simulink model "PMSM_CCSMPC_ClosedLoop"  (R2025b)
settings: Solver=ode3  StartTime=0.0  StopTime=0.4  FixedStep=1e-6  RelTol=1e-3
PreLoadFcn:
  | run('params_pmsm_inverter')
undefined symbols (not defined in the file or in its folder): Iq_max, J, Ld_hat, Lq_hat, pp, PsiPM_hat, Rs_hat, Ts_ctrl, Ts_sim, Vdc
libraries: nesl_utility x13, fl_lib x8, ee_lib x8, simulink x1, slpidlib x1
(part 1 of 2)
settings Model: Creator=Harish  LastModifiedBy=Harish

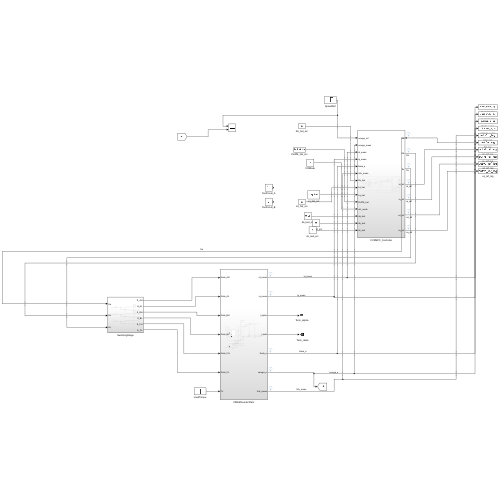
[thumbnail: Simulink's stored preview of the top-level diagram]
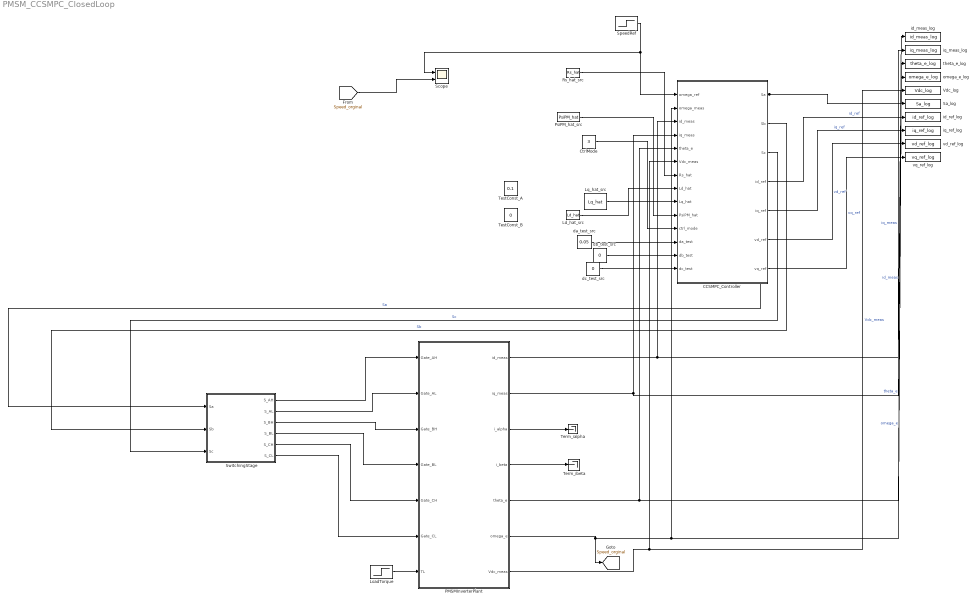
== system PMSM_CCSMPC_ClosedLoop ==
  CCSMPC_Controller : Subsystem
  CtrlMode : Constant  Value=3  OutDataTypeStr=uint8
  Ld_hat_src : Constant  Value=Ld_hat
  LoadTorque : Step  Time=0.25  After=0.05  SampleTime=0
  Lq_hat_src : Constant  Value=Lq_hat
  PMSMInverterPlant : Subsystem
  PsiPM_hat_src : Constant  Value=PsiPM_hat
  Rs_hat_src : Constant  Value=Rs_hat
  Sa_log : ToWorkspace  VariableName=Sa_log  SaveFormat=Timeseries  SampleTime=-1
  Scope : Scope  NumInputPorts=2
      settings: ActiveDisplayYMinimum=-24.999999999999993  ActiveDisplayYMaximum=225
  SpeedRef : Step  Time=0.05  After=200  SampleTime=0
  SwitchingStage : Subsystem
  Term_ialpha : Terminator
  Term_ibeta : Terminator
  TestConst_A : Constant  Value=0.1
  TestConst_B : Constant  Value=0
  Vdc_log : ToWorkspace  VariableName=Vdc_log  SaveFormat=Timeseries  SampleTime=-1
  da_test_src : Constant  Value=0.05
  db_test_src : Constant  Value=0
  dc_test_src : Constant  Value=0
  id_meas_log : ToWorkspace  VariableName=id_meas_log  SaveFormat=Timeseries  SampleTime=-1
  id_ref_log : ToWorkspace  VariableName=id_ref_log  SaveFormat=Timeseries  SampleTime=-1
  iq_meas_log : ToWorkspace  VariableName=iq_meas_log  SaveFormat=Timeseries  SampleTime=-1
  iq_ref_log : ToWorkspace  VariableName=iq_ref_log  SaveFormat=Timeseries  SampleTime=-1
  omega_e_log : ToWorkspace  VariableName=omega_e_log  SaveFormat=Timeseries  SampleTime=-1
  theta_e_log : ToWorkspace  VariableName=theta_e_log  SaveFormat=Timeseries  SampleTime=-1
  vd_ref_log : ToWorkspace  VariableName=vd_ref_log  SaveFormat=Timeseries  SampleTime=-1
  vq_ref_log : ToWorkspace  VariableName=vq_ref_log  SaveFormat=Timeseries  SampleTime=-1
  tag scope: Speed_orginal=global
  wires:
  SpeedRef/1 -> Scope/1, CCSMPC_Controller/1(omega_ref)
  Rs_hat_src/1 -> CCSMPC_Controller/7(Rs_hat)
  Ld_hat_src/1 -> CCSMPC_Controller/8(Ld_hat)
  Lq_hat_src/1 -> CCSMPC_Controller/9(Lq_hat)
  PsiPM_hat_src/1 -> CCSMPC_Controller/10(PsiPM_hat)
  CtrlMode/1 -> CCSMPC_Controller/11(ctrl_mode)
  PMSMInverterPlant/6(omega_e) -> [Speed_orginal], CCSMPC_Controller/2(omega_meas), omega_e_log/1  "omega_e"
  PMSMInverterPlant/1(id_meas) -> id_meas_log/1, CCSMPC_Controller/3(id_meas)  "id_meas"
  PMSMInverterPlant/2(iq_meas) -> iq_meas_log/1, CCSMPC_Controller/4(iq_meas)  "iq_meas"
  PMSMInverterPlant/5(theta_e) -> theta_e_log/1, CCSMPC_Controller/5(theta_e)  "theta_e"
  PMSMInverterPlant/7(Vdc_meas) -> CCSMPC_Controller/6(Vdc_meas), Vdc_log/1  "Vdc_meas"
  CCSMPC_Controller/1(Sa) -> SwitchingStage/1(Sa), Sa_log/1  "Sa"
  CCSMPC_Controller/2(Sb) -> SwitchingStage/2(Sb)  "Sb"
  CCSMPC_Controller/3(Sc) -> SwitchingStage/3(Sc)  "Sc"
  SwitchingStage/1(S_AH) -> PMSMInverterPlant/1(Gate_AH)
  SwitchingStage/2(S_AL) -> PMSMInverterPlant/2(Gate_AL)
  SwitchingStage/3(S_BH) -> PMSMInverterPlant/3(Gate_BH)
  SwitchingStage/4(S_BL) -> PMSMInverterPlant/4(Gate_BL)
  SwitchingStage/5(S_CH) -> PMSMInverterPlant/5(Gate_CH)
  SwitchingStage/6(S_CL) -> PMSMInverterPlant/6(Gate_CL)
  LoadTorque/1 -> PMSMInverterPlant/7(TL)
  CCSMPC_Controller/4(id_ref) -> id_ref_log/1  "id_ref"
  CCSMPC_Controller/5(iq_ref) -> iq_ref_log/1  "iq_ref"
  CCSMPC_Controller/6(vd_ref) -> vd_ref_log/1  "vd_ref"
  CCSMPC_Controller/7(vq_ref) -> vq_ref_log/1  "vq_ref"
  PMSMInverterPlant/3(i_alpha) -> Term_ialpha/1
  PMSMInverterPlant/4(i_beta) -> Term_ibeta/1
  db_test_src/1 -> CCSMPC_Controller/13(db_test)
  dc_test_src/1 -> CCSMPC_Controller/14(dc_test)
  da_test_src/1 -> CCSMPC_Controller/12(da_test)
  [Speed_orginal] -> Scope/2

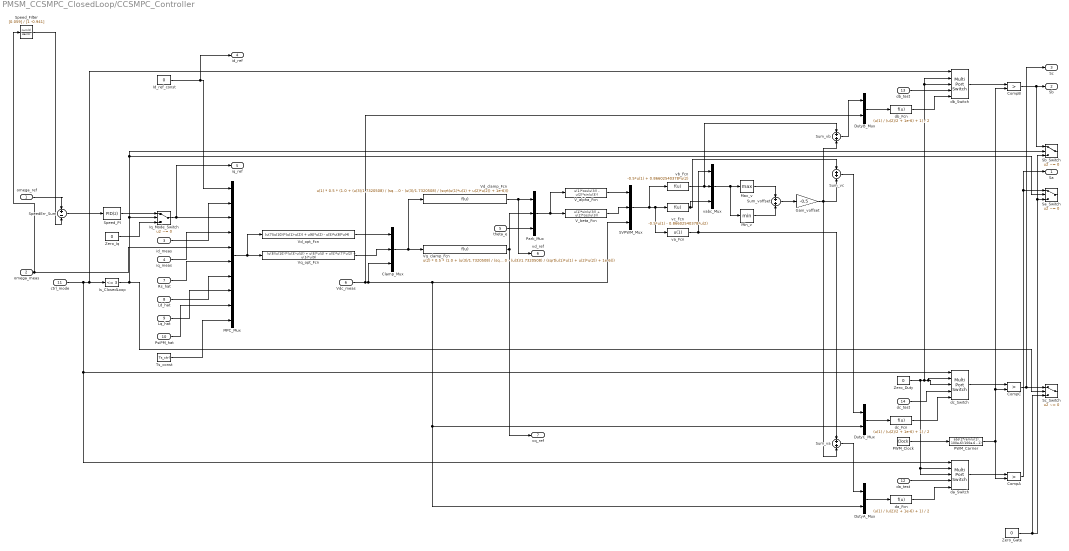
== system PMSM_CCSMPC_ClosedLoop/CCSMPC_Controller ==
  omega_ref : Inport  SampleTime=Ts_ctrl
  omega_meas : Inport  Port=2  SampleTime=Ts_ctrl
  id_meas : Inport  Port=3  SampleTime=Ts_ctrl
  iq_meas : Inport  Port=4  SampleTime=Ts_ctrl
  theta_e : Inport  Port=5  SampleTime=Ts_ctrl
  Vdc_meas : Inport  Port=6  SampleTime=Ts_ctrl
  Rs_hat : Inport  Port=7  SampleTime=Ts_ctrl
  Ld_hat : Inport  Port=8  SampleTime=Ts_ctrl
  Lq_hat : Inport  Port=9  SampleTime=Ts_ctrl
  PsiPM_hat : Inport  Port=10  SampleTime=Ts_ctrl
  ctrl_mode : Inport  Port=11  SampleTime=Ts_ctrl
  da_test : Inport  Port=12
  db_test : Inport  Port=13
  dc_test : Inport  Port=14
  Clamp_Mux : Mux  Inputs=3
  CompA : RelationalOperator  Operator=>  OutDataTypeStr=boolean  SampleTime=Ts_sim  RndMeth=Simplest  InputSameDT=off
  CompB : RelationalOperator  Operator=>  OutDataTypeStr=boolean  SampleTime=Ts_sim  RndMeth=Simplest  InputSameDT=off
  CompC : RelationalOperator  Operator=>  OutDataTypeStr=boolean  SampleTime=Ts_sim  RndMeth=Simplest  InputSameDT=off
  DutyA_Mux : Mux  Inputs=2
  DutyB_Mux : Mux  Inputs=2
  DutyC_Mux : Mux  Inputs=2
  Gain_voffset : Gain  Gain=-0.5
  Id_ref_const : Constant  Value=0  SampleTime=Ts_ctrl
  Iq_Mode_Switch : Switch  Criteria=u2 ~= 0  SaturateOnIntegerOverflow=off  InputSameDT=off
  Is_ClosedLoop : simulink/Logic and Bit Operations/Compare To Constant  relop=<=  const=3  OutDataTypeStr=boolean
  MPC_Mux : Mux  Inputs=10
  Max_v : MinMax  Function=max
  Min_v : MinMax
  PWM_Carrier : Fcn  Expr=abs(2*rem(u(1), 100e-6)/100e-6 - 1)
  PWM_Clock : DigitalClock  SampleTime=Ts_sim
  Park_Mux : Mux  Inputs=3
  SVPWM_Mux : Mux  Inputs=3
  Sa_Switch : Switch  Criteria=u2 ~= 0  SaturateOnIntegerOverflow=off  InputSameDT=off
  Sb_Switch : Switch  Criteria=u2 ~= 0  SaturateOnIntegerOverflow=off  InputSameDT=off
  Sc_Switch : Switch  Criteria=u2 ~= 0  SaturateOnIntegerOverflow=off  InputSameDT=off
  SpeedErr_Sum : Sum  Inputs=+-
  Speed_Filter : DiscreteFilter  Numerator=[0.059]  Denominator=[1 -0.941]  SampleTime=Ts_ctrl
  Speed_PI : slpidlib/PID Controller  Controller=PID  Form=Parallel  TimeDomain=Discrete-time  UseExternalTs=off  SampleTime=Ts_ctrl  IntegratorMethod=Forward Euler  FilterMethod=Forward Euler  ControllerParametersSource=internal  P=0.01  I=1.5  UseKiTs=off  D=0  UseExternalDerivativeSource=off  N=100  UseFilter=on  TunerSelectOption=Transfer Function Based (PID Tuner App)  InitialConditionSource=internal  InitialConditionForIntegrator=0  InitialConditionForFilter=0  DifferentiatorICPrevScaledInput=0  ExternalReset=none  TrackingMode=off  Kt=1  LimitOutput=on  SatLimitsSource=internal  UpperSaturationLimit=Iq_max  LowerSaturationLimit=-Iq_max  LinearizeAsGain=on  AntiWindupMode=clamping  Kb=1  LimitIntegrator=off  UpperIntegratorSaturationLimit=inf  LowerIntegratorSaturationLimit=-inf  POutMin=[]  POutMax=[]  IOutMin=[]  IOutMax=[]  DOutMin=[]  DOutMax=[]  NOutMin=[]  NOutMax=[]  SumOutMin=[]  SumOutMax=[]  SaturationOutMin=[]  SaturationOutMax=[]  PParamMin=[]  PParamMax=[]  IParamMin=[]  IParamMax=[]  DParamMin=[]  DParamMax=[]  NParamMin=[]  NParamMax=[]  KbParamMin=[]  KbParamMax=[]  KtParamMin=[]  KtParamMax=[]  KbOutMin=[]  KbOutMax=[]  KtOutMin=[]  KtOutMax=[]  IntegratorOutMin=[]  IntegratorOutMax=[]  FilterOutMin=[]  FilterOutMax=[]  SumI1OutMin=[]  SumI1OutMax=[]  SumI2OutMin=[]  SumI2OutMax=[]  SumI3OutMin=[]  SumI3OutMax=[]  SumI4OutMin=[]  SumI4OutMax=[]  SumDOutMin=[]  SumDOutMax=[]  DifferentiatorOutMin=[]  DifferentiatorOutMax=[]  FilterDiffOutCoefMin=[]  FilterDiffOutCoefMax=[]  ReciprocalOutMin=[]  ReciprocalOutMax=[]  SumDenOutMin=[]  SumDenOutMax=[]  SumNumOutMin=[]  SumNumOutMax=[]  DivideOutMin=[]  DivideOutMax=[]  UdiffTsProdOutMin=[]  UdiffTsProdOutMax=[]  NTsProdOutMin=[]  NTsProdOutMax=[]  UintegralTsProdOutMin=[]  UintegralTsProdOutMax=[]  UngainTsProdOutMin=[]  UngainTsProdOutMax=[]  ClampingZeroOutDataTypeStr=Inherit: Inherit via back propagation  ClampingZeroOutMin=[]  ClampingZeroOutMax=[]  FilterDenConstantOutDataTypeStr=Inherit: Inherit via back propagation  FilterDenConstantOutMin=[]  FilterDenConstantOutMax=[]  PCopyOutDataTypeStr=Inherit: Inherit via back propagation  PCopyOutMin=[]  PCopyOutMax=[]  NCopyOutDataTypeStr=Inherit: Inherit via back propagation  NCopyOutMin=[]  NCopyOutMax=[]  IntegratorContinuousStateAttributes=''  IntegratorStateMustResolveToSignalObject=off  IntegratorRTWStateStorageClass=Auto  FilterContinuousStateAttributes=''  FilterStateMustResolveToSignalObject=off  FilterRTWStateStorageClass=Auto  ParallelPVariant=InternalParameters  IdealPVariant=Disabled  IVariant=InternalParameters  DVariant=InternalParameters  IntegratorVariant=Discrete  SatVariant=Enabled  AWVariant=DiscClampingParallel  PCopyVariant=Disabled  TRVariant=Disabled  FdbkBlocksVariant=Forward  IdealPFdbkVariant=Disabled  SatFdbkVariant=Disabled  DerivativeFilterVariant=ForwardEulerFilter  NVariant=InternalParameters  NCopyVariant=Disabled  FilterICVariant=InternalICsFilter  IntegratorICVariant=InternalICs  ExternalResetVariant=Disabled  TRSumVariant=Passthrough  SumFdbkVariant=Disabled  SumVariant=Sum_PID  TsampFilterVariant=InternalTs  TsampNgainVariant=Passthrough  TsampIntegralVariant=Disabled_SignalSpec  ExternalSaturationOutDataTypeStr=Inherit: Same as second input  DerivativeSourceVariant=ErrorSignal  PreIntVariant=InternalPreInt
  Sum_va : Sum
  Sum_vb : Sum
  Sum_vc : Sum
  Sum_voffset : Sum
  Ts_const : Constant  Value=Ts_ctrl  SampleTime=Ts_ctrl
  V_alpha_Fcn : Fcn  Expr=u(1)*cos(u(3)) - u(2)*sin(u(3))
  V_beta_Fcn : Fcn  Expr=u(1)*sin(u(3)) + u(2)*cos(u(3))
  Vd_clamp_Fcn : Fcn  Expr=u(1) * 0.5 * (1.0 + (u(3)/1.7320508) / (sqrt(u(1)*u(1) + u(2)*u(2)) + 1e-6) - abs(1.0 - (u(3)/1.7320508) / (sqrt(u(1)*u(1) + u(2)*u(2)) + 1e-6)))
  Vd_opt_Fcn : Fcn  Expr=(u(7)/u(10))*(u(1)-u(2)) + u(6)*u(2) - u(5)*u(8)*u(4)
  Vq_clamp_Fcn : Fcn  Expr=u(2) * 0.5 * (1.0 + (u(3)/1.7320508) / (sqrt(u(1)*u(1) + u(2)*u(2)) + 1e-6) - abs(1.0 - (u(3)/1.7320508) / (sqrt(u(1)*u(1) + u(2)*u(2)) + 1e-6)))
  Vq_opt_Fcn : Fcn  Expr=(u(8)/u(10))*(u(3)-u(4)) + u(6)*u(4) + u(5)*u(7)*u(2) + u(5)*u(9)
  Zero_Duty : Constant  Value=0
  Zero_Gate : Constant  Value=0  OutDataTypeStr=boolean  SampleTime=Ts_ctrl
  Zero_Iq : Constant  Value=0  SampleTime=Ts_ctrl
  da_Fcn : Fcn  Expr=(u(1) / (u(2)/2 + 1e-6) + 1) / 2
  da_Switch : MultiPortSwitch  DataPortOrder=Zero-based contiguous  Inputs=4  zeroidx=on  SaturateOnIntegerOverflow=off  InputSameDT=off
  db_Fcn : Fcn  Expr=(u(1) / (u(2)/2 + 1e-6) + 1) / 2
  db_Switch : MultiPortSwitch  DataPortOrder=Zero-based contiguous  Inputs=4  zeroidx=on  SaturateOnIntegerOverflow=off  InputSameDT=off
  dc_Fcn : Fcn  Expr=(u(1) / (u(2)/2 + 1e-6) + 1) / 2
  dc_Switch : MultiPortSwitch  DataPortOrder=Zero-based contiguous  Inputs=4  zeroidx=on  SaturateOnIntegerOverflow=off  InputSameDT=off
  va_Fcn : Fcn  Expr=u(1)
  vabc_Mux : Mux  Inputs=3
  vb_Fcn : Fcn  Expr=-0.5*u(1) + 0.86602540378*u(2)
  vc_Fcn : Fcn  Expr=-0.5*u(1) - 0.86602540378*u(2)
  Sa : Outport  SampleTime=Ts_ctrl
  Sb : Outport  Port=2  SampleTime=Ts_ctrl
  Sc : Outport  Port=3  SampleTime=Ts_ctrl
  id_ref : Outport  Port=4  SampleTime=Ts_ctrl
  iq_ref : Outport  Port=5  SampleTime=Ts_ctrl
  vd_ref : Outport  Port=6  SampleTime=Ts_ctrl
  vq_ref : Outport  Port=7  SampleTime=Ts_ctrl
  wires:
  ctrl_mode/1 -> dc_Switch/1, da_Switch/1, db_Switch/1, Is_ClosedLoop/1
  omega_ref/1 -> SpeedErr_Sum/1
  Sum_va/1 -> DutyA_Mux/1
  Sum_vb/1 -> DutyB_Mux/1
  Speed_PI/1 -> Iq_Mode_Switch/1
  SpeedErr_Sum/1 -> Speed_PI/1
  Zero_Iq/1 -> Iq_Mode_Switch/3
  Id_ref_const/1 -> id_ref/1, MPC_Mux/1
  Vd_opt_Fcn/1 -> Clamp_Mux/1
  Is_ClosedLoop/1 -> Sa_Switch/2, Sb_Switch/2, Iq_Mode_Switch/2, Sc_Switch/2
  db_Fcn/1 -> db_Switch/5
  DutyC_Mux/1 -> dc_Fcn/1
  DutyB_Mux/1 -> db_Fcn/1
  Iq_Mode_Switch/1 -> iq_ref/1, MPC_Mux/3
  Zero_Gate/1 -> Sa_Switch/3, Sb_Switch/3, Sc_Switch/3
  da_test/1 -> da_Switch/4
  Vq_opt_Fcn/1 -> Clamp_Mux/2
  MPC_Mux/1 -> Vd_opt_Fcn/1, Vq_opt_Fcn/1
  id_meas/1 -> MPC_Mux/2
  iq_meas/1 -> MPC_Mux/4
  db_test/1 -> db_Switch/4
  Rs_hat/1 -> MPC_Mux/6
  CompC/1 -> Sc_Switch/1, Sc/1
  CompB/1 -> Sb_Switch/1, Sb/1
  dc_Switch/1 -> CompC/1
  Ld_hat/1 -> MPC_Mux/7
  dc_Fcn/1 -> dc_Switch/5
  theta_e/1 -> Park_Mux/3
  Lq_hat/1 -> MPC_Mux/8
  dc_test/1 -> dc_Switch/4
  DutyA_Mux/1 -> da_Fcn/1
  PsiPM_hat/1 -> MPC_Mux/9
  Ts_const/1 -> MPC_Mux/10
  Vdc_meas/1 -> DutyC_Mux/2, DutyA_Mux/2, SVPWM_Mux/3, Clamp_Mux/3, DutyB_Mux/2
  Clamp_Mux/1 -> Vd_clamp_Fcn/1, Vq_clamp_Fcn/1
  Max_v/1 -> Sum_voffset/1
  Vd_clamp_Fcn/1 -> vd_ref/1, Park_Mux/1
  Vq_clamp_Fcn/1 -> vq_ref/1, Park_Mux/2
  PWM_Carrier/1 -> CompB/2, CompC/2, CompA/2
  Park_Mux/1 -> V_alpha_Fcn/1, V_beta_Fcn/1
  V_alpha_Fcn/1 -> SVPWM_Mux/1
  Sum_vc/1 -> DutyC_Mux/1
  Sum_voffset/1 -> Gain_voffset/1
  V_beta_Fcn/1 -> SVPWM_Mux/2
  SVPWM_Mux/1 -> vc_Fcn/1, va_Fcn/1, vb_Fcn/1
  CompA/1 -> Sa_Switch/1, Sa/1
  va_Fcn/1 -> Sum_va/1, vabc_Mux/1
  vb_Fcn/1 -> Sum_vb/1, vabc_Mux/2
  vc_Fcn/1 -> Sum_vc/1, vabc_Mux/3
  vabc_Mux/1 -> Min_v/1, Max_v/1
  Min_v/1 -> Sum_voffset/2
  Gain_voffset/1 -> Sum_vb/2, Sum_vc/2, Sum_va/2
  Zero_Duty/1 -> da_Switch/2, da_Switch/3, dc_Switch/2, dc_Switch/3, db_Switch/2, db_Switch/3
  PWM_Clock/1 -> PWM_Carrier/1
  da_Fcn/1 -> da_Switch/5
  db_Switch/1 -> CompB/1
  da_Switch/1 -> CompA/1
  omega_meas/1 -> Speed_Filter/1, MPC_Mux/5
  Speed_Filter/1 -> SpeedErr_Sum/2

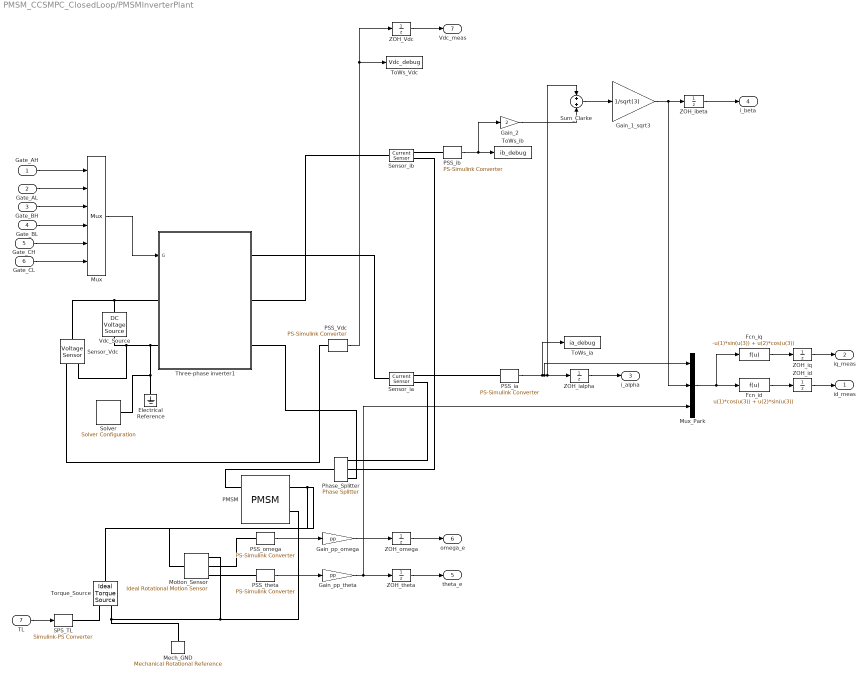
== system PMSM_CCSMPC_ClosedLoop/PMSMInverterPlant ==
  Gate_AH : Inport
  Gate_AL : Inport  Port=2
  Gate_BH : Inport  Port=3
  Gate_BL : Inport  Port=4
  Gate_CH : Inport  Port=5
  Gate_CL : Inport  Port=6
  TL : Inport  Port=7
  Electrical Reference : fl_lib/Electrical/Electrical Elements/Electrical Reference
  Fcn_id : Fcn  Expr=u(1)*cos(u(3)) + u(2)*sin(u(3))
  Fcn_iq : Fcn  Expr=-u(1)*sin(u(3)) + u(2)*cos(u(3))
  Gain_1_sqrt3 : Gain  Gain=1/sqrt(3)
  Gain_2 : Gain  Gain=2
  Gain_pp_omega : Gain  Gain=pp
  Gain_pp_theta : Gain  Gain=pp
  Mech_GND : fl_lib/Mechanical/Rotational Elements/Mechanical Rotational Reference
  Motion_Sensor : fl_lib/Mechanical/Mechanical Sensors/Ideal Rotational Motion Sensor  reference=foundation.enum.MeasurementReference.difference  acceleration_port=false  velocity_port=true  position_port=true  wrap_angle=false  offset=0 rad
  Mux : Mux  Inputs=6
  Mux_Park : Mux  Inputs=3
  PMSM : ee_lib/Electromechanical/Permanent Magnet/PMSM  port_option=1  winding_type=ee.enum.electromech.statorconfiguration.wye  machine_param=ee.enum.pmsm.parameterization.constant  nPolePairs=pp  pmflux_param=ee.enum.pmflux.fluxlinkage  pm_flux_linkage=PsiPM Wb  torque_constant=0.18 N*m/A  back_emf_constant=0.18 V*s/rad  stator_param=1  Ld=Ld H  Lq=Lq H  idVec=[-200, 0, 200] A  iqVec=[-200, 0, 200] A  LdMatrix=0.0002 * ones(3, 3) H  LqMatrix=0.0002 * ones(3, 3) H  PmMatrix=0.1 * ones(3, 3) Wb  ktMatrix=0.18 * ones(3, 3) N*m/A  keMatrix=0.18 * ones(3, 3) V*s/rad  L0=0.00016 H  Ls=0.0002 H  Lm=-0.00002 H  Ms=0.00002 H  Rs=Rs Ohm  zero_sequence=ee.enum.park.zerosequence.include  axes_param=ee.enum.rotorangle.daxis  loss_param=ee.enum.ironloss.none  losses_oc=[0, 0, 0] W  losses_sc=[0, 0, 0] W  f_losses=60 Hz  Isc_losses=95 A  J=J kg*m^2  lam=B_fric N*m*s/rad  i_d_specify=off  i_d_priority=None  i_d=0 A  i_d_nominal_specify=off  i_d_nominal_value=1  i_d_nominal_unit=A  i_q_specify=off  i_q_priority=None  i_q=0 A  i_q_nominal_specify=off  i_q_nominal_value=1  i_q_nominal_unit=A  torque_specify=off  torque_priority=None  torque=0 N*m  torque_nominal_specify=off  torque_nominal_value=1  torque_nominal_unit=N*m  angular_velocity_specify=off  angular_velocity_priority=High  angular_velocity=0 rpm  angular_velocity_nominal_specify=off  angular_velocity_nominal_value=1  angular_velocity_nominal_unit=rpm  angular_position_specify=off  angular_position_priority=High  angular_position=0 deg  angular_position_nominal_specify=off  angular_position_nominal_value=1  angular_position_nominal_unit=deg  alpha=3.93e-3 1/K  alpha_flux=-0.001 1/K  Tmeas=298.15 K  stator_thermal_mass=100 J/K  rotor_thermal_mass=200 J/K  Rm_percent_rotor=90  Rd_percent_rotor=30  temperatureA_specify=off  temperatureA_priority=High  temperatureA=25 degC  temperatureA_nominal_specify=off  temperatureA_nominal_value=1  temperatureA_nominal_unit=degC  temperatureB_specify=off  temperatureB_priority=High  temperatureB=25 degC  temperatureB_nominal_specify=off  temperatureB_nominal_value=1  temperatureB_nominal_unit=degC  temperatureC_specify=off  temperatureC_priority=High  temperatureC=25 degC  temperatureC_nominal_specify=off  temperatureC_nominal_value=1  temperatureC_nominal_unit=degC  temperatureR_specify=off  temperatureR_priority=High  temperatureR=25 degC  temperatureR_nominal_specify=off  temperatureR_nominal_value=1  temperatureR_nominal_unit=degC
      settings: InternalSimscapePortConfiguration="{\"Bottom\":[],\"Left\":[{\"id\":\"N\",\"label\":\"~\",\"type\":\"foundation.electrical.three_phase\"},{\"id\":\"n\",\"label\":\"n\",\"type\":\"foundation.electrical.electrical\"}],\"Right\":[{\"id\":\"R\",\"label\":\"R\",\"type\":\"foundation.mechanical.rotational.rotational\"},{\"id\":\"C\",\"label\":\"C\",\"type\":\"foundation.mechanical.rotational.rotational\"}],\"Top\":[]}"
  PSS_Vdc : nesl_utility/PS-Simulink Converter  PhysicalDomain=network_engine_domain  SubClassName=ps_output  LeftPortType=input  RightPortType=output  PseudoPeriodic=off  Frequencies=[]  VectorFormat=inherit  Unit=inherit  AffineConversion=off
  PSS_ia : nesl_utility/PS-Simulink Converter  PhysicalDomain=network_engine_domain  SubClassName=ps_output  LeftPortType=input  RightPortType=output  PseudoPeriodic=off  Frequencies=[]  VectorFormat=inherit  Unit=inherit  AffineConversion=off
  PSS_ib : nesl_utility/PS-Simulink Converter  PhysicalDomain=network_engine_domain  SubClassName=ps_output  LeftPortType=input  RightPortType=output  PseudoPeriodic=off  Frequencies=[]  VectorFormat=inherit  Unit=inherit  AffineConversion=off
  PSS_omega : nesl_utility/PS-Simulink Converter  PhysicalDomain=network_engine_domain  SubClassName=ps_output  LeftPortType=input  RightPortType=output  PseudoPeriodic=off  Frequencies=[]  VectorFormat=inherit  Unit=inherit  AffineConversion=off
  PSS_theta : nesl_utility/PS-Simulink Converter  PhysicalDomain=network_engine_domain  SubClassName=ps_output  LeftPortType=input  RightPortType=output  PseudoPeriodic=off  Frequencies=[]  VectorFormat=inherit  Unit=inherit  AffineConversion=off
  Phase_Splitter : ee_lib/Connectors & References/Phase Splitter
  SPS_TL : nesl_utility/Simulink-PS Converter  PhysicalDomain=network_engine_domain  SubClassName=ps_input  LeftPortType=input  RightPortType=output  PseudoPeriodic=off  Frequencies=[]  NoiseDistribution=none  NoiseParameters=[]  Unit=1  AffineConversion=off  FilteringAndDerivatives=filter  SimscapeFilterOrder=1  InputFilterTimeConstant=0.001  UdotUserProvided=0
  Sensor_Vdc : fl_lib/Electrical/Electrical Sensors/Voltage Sensor
  Sensor_ia : fl_lib/Electrical/Electrical Sensors/Current Sensor
  Sensor_ib : fl_lib/Electrical/Electrical Sensors/Current Sensor
  Solver : nesl_utility/Solver Configuration  PhysicalDomain=network_engine_domain  SubClassName=solver  LeftPortType=input  RightPortType=generic  Tones=[]  Harmonics=[]  SimulateNoise=off  Profile=off  UseLocalSampling=off  EnableSwitchedLinearOptims=on  FrequencyDomain=off  UseCCode=off  RelTol=0.001  AbsTol=0.001  MinStep=1e-09  ToWorkspace=off  RevertToSquareIcSolve=off  NumHomotopyIterations=100  PhasorMode=off  PhasorModeNumHarmonics=1  ConsistencySolver=NEWTON_XTOL_AFTER_FTOL  IndexReductionMethod=DerivativeReplacement  DoDC=off  ResidualTolerance=1e-09  ConsistencyTolSource=GLOBAL  ConsistencyAbsTol=0.001  ConsistencyRelTol=0.001  ConsistencyTolFactor=0.001  UseLocalSolver=on  LocalSolverChoice=NE_BACKWARD_EULER_ADVANCER  ResolveIndetEquations=on  FunctionEvalNumThread=1  LocalSolverSampleTime=Ts_sim  DoFixedCost=off  MaxNonlinIter=3  MaxModeIter=2  ComputeImpulses=off  ImpulseIterations=2  LinearAlgebra=auto  LinearAlgebraNumThread=0  EquationFormulation=NE_TIME_EF  DelaysMemoryBudget=1024  AutomaticFiltering=on  FilteringTimeConstant=0.001  PartitionStorageMethod=AS_NEEDED  PartitionMemoryBudget=1024  PartitionMethod=ROBUST  MultibodyUseLocalSolver=off  MultibodyLocalSolverChoice=ODE1  MultibodyLocalSolverSampleTime=0.001
  Sum_Clarke : Sum
  Three-phase inverter1 : Subsystem
      mask Display: image('Inverter.jpg');
  ToWs_Vdc : ToWorkspace  VariableName=Vdc_debug  SampleTime=-1
  ToWs_ia : ToWorkspace  VariableName=ia_debug  SampleTime=-1
  ToWs_ib : ToWorkspace  VariableName=ib_debug  SampleTime=-1
  Torque_Source : fl_lib/Mechanical/Mechanical Sources/Ideal Torque Source
  Vdc_Source : fl_lib/Electrical/Electrical Sources/DC Voltage Source  v0=48 V
  ZOH_Vdc : UnitDelay  InitialCondition=Vdc  SampleTime=Ts_ctrl  HasFrameUpgradeWarning=on
  ZOH_ialpha : UnitDelay  SampleTime=Ts_ctrl  HasFrameUpgradeWarning=on
  ZOH_ibeta : UnitDelay  SampleTime=Ts_ctrl  HasFrameUpgradeWarning=on
  ZOH_id : UnitDelay  SampleTime=Ts_ctrl  HasFrameUpgradeWarning=on
  ZOH_iq : UnitDelay  SampleTime=Ts_ctrl  HasFrameUpgradeWarning=on
  ZOH_omega : UnitDelay  SampleTime=Ts_ctrl  HasFrameUpgradeWarning=on
  ZOH_theta : UnitDelay  SampleTime=Ts_ctrl  HasFrameUpgradeWarning=on
  id_meas : Outport
  iq_meas : Outport  Port=2
  i_alpha : Outport  Port=3
  i_beta : Outport  Port=4
  theta_e : Outport  Port=5
  omega_e : Outport  Port=6
  Vdc_meas : Outport  Port=7
  wires:
  TL/1 -> SPS_TL/1
  Mux_Park/1 -> Fcn_iq/1, Fcn_id/1
  PSS_omega/1 -> Gain_pp_omega/1
  Fcn_iq/1 -> ZOH_iq/1
  Gain_2/1 -> Sum_Clarke/2
  PSS_theta/1 -> Gain_pp_theta/1
  Fcn_id/1 -> ZOH_id/1
  Gain_1_sqrt3/1 -> ZOH_ibeta/1, Mux_Park/2
  PSS_Vdc/1 -> ToWs_Vdc/1, ZOH_Vdc/1
  PSS_ia/1 -> ZOH_ialpha/1, Sum_Clarke/1, Mux_Park/1, ToWs_ia/1
  Gain_pp_omega/1 -> ZOH_omega/1
  Gain_pp_theta/1 -> ZOH_theta/1, Mux_Park/3
  ZOH_Vdc/1 -> Vdc_meas/1
  ZOH_omega/1 -> omega_e/1
  ZOH_theta/1 -> theta_e/1
  PSS_ib/1 -> Gain_2/1, ToWs_ib/1
  Sum_Clarke/1 -> Gain_1_sqrt3/1
  ZOH_ialpha/1 -> i_alpha/1
  ZOH_ibeta/1 -> i_beta/1
  ZOH_iq/1 -> iq_meas/1
  ZOH_id/1 -> id_meas/1
  Gate_AH/1 -> Mux/1
  Gate_AL/1 -> Mux/2
  Gate_BH/1 -> Mux/3
  Gate_BL/1 -> Mux/4
  Gate_CH/1 -> Mux/5
  Gate_CL/1 -> Mux/6
  Mux/1 -> Three-phase inverter1/1(G)
  connections:
  SPS_TL/RConn1 -- Torque_Source/RConn1
  Torque_Source/RConn2 -- Motion_Sensor/RConn1 -- PMSM/RConn2 -- Mech_GND/LConn1
  Motion_Sensor/LConn1 -- PMSM/RConn1 -- Torque_Source/LConn1
  Phase_Splitter/LConn1 -- PMSM/LConn1
  Motion_Sensor/RConn2 -- PSS_omega/LConn1
  Motion_Sensor/RConn3 -- PSS_theta/LConn1
  Sensor_ib/RConn1 -- PSS_ib/LConn1
  Sensor_Vdc/RConn1 -- PSS_Vdc/LConn1
  Sensor_ib/RConn2 -- Phase_Splitter/RConn2
  Sensor_ia/RConn1 -- PSS_ia/LConn1
  Sensor_ia/RConn2 -- Phase_Splitter/RConn1
  Vdc_Source/LConn1 -- Sensor_Vdc/LConn1 -- Three-phase inverter1/LConn1
  Vdc_Source/RConn1 -- Sensor_Vdc/RConn2 -- Solver/RConn1 -- Electrical Reference/LConn1 -- Three-phase inverter1/LConn2
  Sensor_ia/LConn1 -- Three-phase inverter1/RConn1
  Three-phase inverter1/RConn2 -- Sensor_ib/LConn1
  Three-phase inverter1/RConn3 -- Phase_Splitter/RConn3

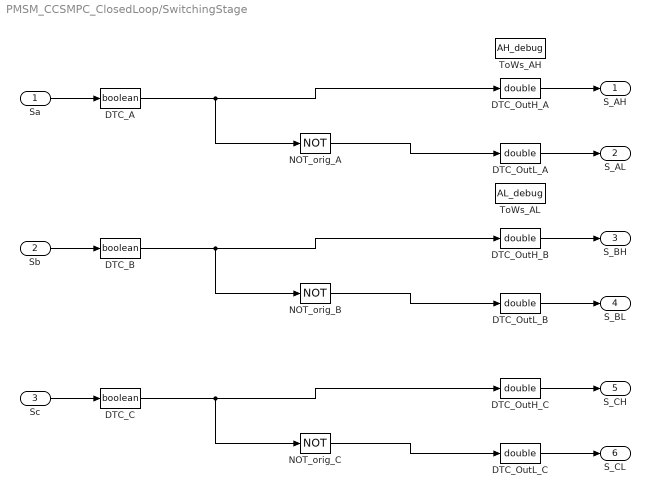
== system PMSM_CCSMPC_ClosedLoop/SwitchingStage ==
  Sa : Inport  SampleTime=Ts_sim
  Sb : Inport  Port=2  SampleTime=Ts_sim
  Sc : Inport  Port=3  SampleTime=Ts_sim
  DTC_A : DataTypeConversion  OutDataTypeStr=boolean  SampleTime=Ts_sim  SaturateOnIntegerOverflow=off  RndMeth=Floor
  DTC_B : DataTypeConversion  OutDataTypeStr=boolean  SampleTime=Ts_sim  SaturateOnIntegerOverflow=off  RndMeth=Floor
  DTC_C : DataTypeConversion  OutDataTypeStr=boolean  SampleTime=Ts_sim  SaturateOnIntegerOverflow=off  RndMeth=Floor
  DTC_OutH_A : DataTypeConversion  OutDataTypeStr=double  SampleTime=Ts_sim  SaturateOnIntegerOverflow=off  RndMeth=Floor
  DTC_OutH_B : DataTypeConversion  OutDataTypeStr=double  SampleTime=Ts_sim  SaturateOnIntegerOverflow=off  RndMeth=Floor
  DTC_OutH_C : DataTypeConversion  OutDataTypeStr=double  SampleTime=Ts_sim  SaturateOnIntegerOverflow=off  RndMeth=Floor
  DTC_OutL_A : DataTypeConversion  OutDataTypeStr=double  SampleTime=Ts_sim  SaturateOnIntegerOverflow=off  RndMeth=Floor
  DTC_OutL_B : DataTypeConversion  OutDataTypeStr=double  SampleTime=Ts_sim  SaturateOnIntegerOverflow=off  RndMeth=Floor
  DTC_OutL_C : DataTypeConversion  OutDataTypeStr=double  SampleTime=Ts_sim  SaturateOnIntegerOverflow=off  RndMeth=Floor
  NOT_orig_A : Logic  Operator=NOT  AllPortsSameDT=off  OutDataTypeStr=boolean  SampleTime=Ts_sim
  NOT_orig_B : Logic  Operator=NOT  AllPortsSameDT=off  OutDataTypeStr=boolean  SampleTime=Ts_sim
  NOT_orig_C : Logic  Operator=NOT  AllPortsSameDT=off  OutDataTypeStr=boolean  SampleTime=Ts_sim
  ToWs_AH : ToWorkspace  VariableName=AH_debug  SaveFormat=Timeseries  SampleTime=-1
  ToWs_AL : ToWorkspace  VariableName=AL_debug  SaveFormat=Timeseries  SampleTime=-1
  S_AH : Outport  SampleTime=Ts_sim
  S_AL : Outport  Port=2  SampleTime=Ts_sim
  S_BH : Outport  Port=3  SampleTime=Ts_sim
  S_BL : Outport  Port=4  SampleTime=Ts_sim
  S_CH : Outport  Port=5  SampleTime=Ts_sim
  S_CL : Outport  Port=6  SampleTime=Ts_sim
  wires:
  Sa/1 -> DTC_A/1
  DTC_A/1 -> DTC_OutH_A/1, NOT_orig_A/1
  NOT_orig_A/1 -> DTC_OutL_A/1
  DTC_OutH_A/1 -> S_AH/1
  DTC_OutL_A/1 -> S_AL/1
  Sb/1 -> DTC_B/1
  DTC_B/1 -> DTC_OutH_B/1, NOT_orig_B/1
  NOT_orig_B/1 -> DTC_OutL_B/1
  DTC_OutH_B/1 -> S_BH/1
  DTC_OutL_B/1 -> S_BL/1
  Sc/1 -> DTC_C/1
  DTC_C/1 -> DTC_OutH_C/1, NOT_orig_C/1
  NOT_orig_C/1 -> DTC_OutL_C/1
  DTC_OutH_C/1 -> S_CH/1
  DTC_OutL_C/1 -> S_CL/1
